simulink model "Final_big_controller"  (R2023b)
settings: Solver=VariableStepAuto  StartTime=0.0  StopTime=20  RelTol=1e-3
model workspace (MAT data in the model file):
  Kp_v = 1.5
  Kp_w = 6
settings Model: Creator=patel  LastModifiedBy=patel

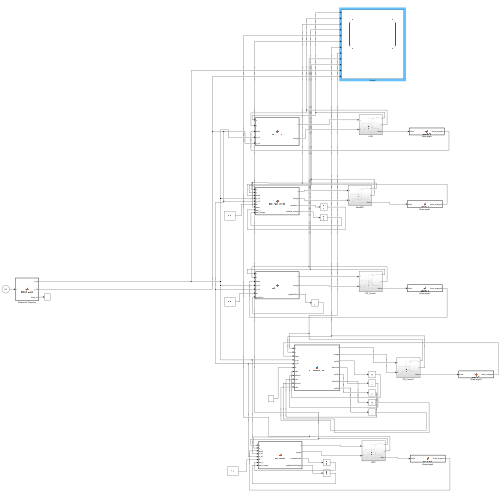
[thumbnail: Simulink's stored preview of the top-level diagram]
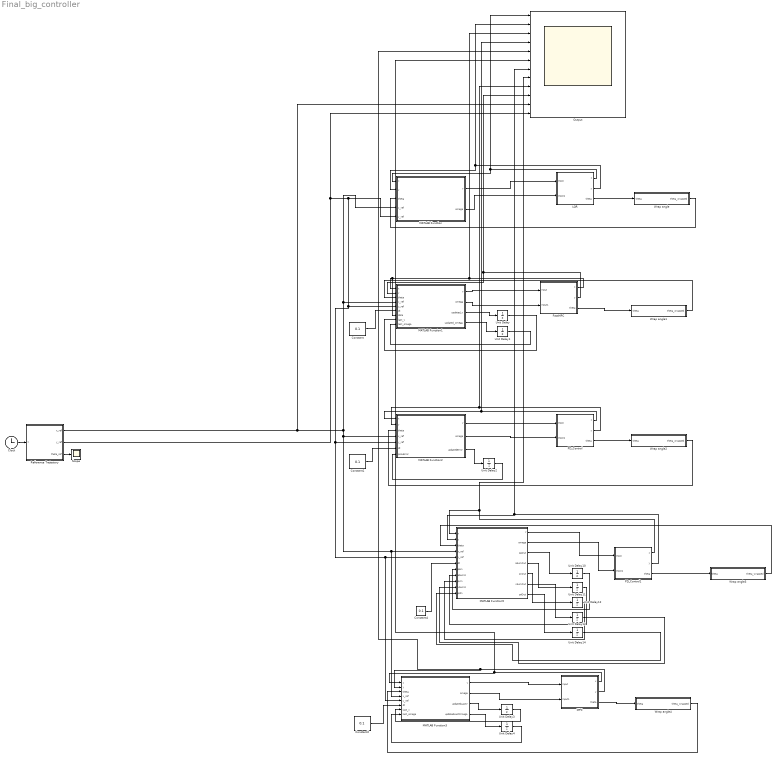
== system Final_big_controller ==
  Clock : Clock
      settings: Decimation=20
  Constant{,1..2,4} (4 alike) : Constant  Value=0.1
  FastMPC : Subsystem
  LQR : Subsystem
  MATLAB Function : MATLAB Function  TreatAsAtomicUnit=on
  MATLAB Function1 : MATLAB Function  TreatAsAtomicUnit=on
  MATLAB Function2 : MATLAB Function  TreatAsAtomicUnit=on
  MATLAB Function3 : MATLAB Function  TreatAsAtomicUnit=on
  MATLAB Function5 : MATLAB Function  TreatAsAtomicUnit=on
  MPC : Subsystem
  Output : Scope  NumInputPorts=12
  PD_Control : Subsystem
  PD_Control1 : Subsystem
  Reference Trajectory : MATLAB Function  TreatAsAtomicUnit=on
  Scope : Scope
  Unit Delay{,1..4,10..14} (10 alike) : UnitDelay  SampleTime=-1  HasFrameUpgradeWarning=on
  Wrap angle : MATLAB Function  TreatAsAtomicUnit=on
  Wrap angle1 : MATLAB Function  TreatAsAtomicUnit=on
  Wrap angle2 : MATLAB Function  TreatAsAtomicUnit=on
  Wrap angle3 : MATLAB Function  TreatAsAtomicUnit=on
  Wrap angle4 : MATLAB Function  TreatAsAtomicUnit=on
  wires:
  Reference Trajectory/3(theta_ref) -> Scope/1
  Clock/1 -> Reference Trajectory/1(t)
  MATLAB Function/2(omega) -> LQR/2(Input1)
  LQR/2(y) -> MATLAB Function/2(y), Output/2
  Wrap angle/1(theta_wrapped) -> MATLAB Function/3(theta)
  LQR/1(x) -> MATLAB Function/1(x), Output/1
  LQR/3(theta) -> Wrap angle/1(theta)
  MATLAB Function/1(v) -> LQR/1(Input)
  MATLAB Function1/4(updated_omega) -> Unit Delay1/1
  MATLAB Function1/3(updated_v) -> Unit Delay/1
  Constant/1 -> MATLAB Function1/6(dt)
  Unit Delay1/1 -> MATLAB Function1/9(last_omega)
  Unit Delay/1 -> MATLAB Function1/8(last_v)
  PD_Control/2(y) -> MATLAB Function2/2(y), Output/9
  MATLAB Function2/1(v) -> PD_Control/1(Input)
  Constant1/1 -> MATLAB Function2/6(dt)
  MATLAB Function2/2(omega) -> PD_Control/2(Input1)
  MATLAB Function2/3(updatedError) -> Unit Delay2/1
  PD_Control/1(x) -> Output/4, MATLAB Function2/1(x)
  Unit Delay2/1 -> MATLAB Function2/7(prevError)
  PD_Control1/1(x) -> MATLAB Function5/1(x), Output/8
  PD_Control1/2(y) -> Output/7, MATLAB Function5/2(y)
  Unit Delay4/1 -> MATLAB Function3/8(last_omega)
  Unit Delay3/1 -> MATLAB Function3/7(last_v)
  Reference Trajectory/2(y_ref) -> Output/12, MATLAB Function3/5(y_ref), MATLAB Function5/5(y_ref), MATLAB Function2/5(y_ref), MATLAB Function1/5(y_ref), MATLAB Function/5(y_ref)
  MPC/1(x) -> Output/6, MATLAB Function3/1(x)
  MPC/3(theta) -> Wrap angle4/1(theta)
  MATLAB Function3/3(updatedLastV) -> Unit Delay3/1
  Wrap angle4/1(theta_wrapped) -> MATLAB Function3/3(theta)
  MATLAB Function3/2(omega) -> MPC/2(Input1)
  Reference Trajectory/1(x_ref) -> Output/11, MATLAB Function/4(x_ref), MATLAB Function1/4(x_ref), MATLAB Function3/4(x_ref), MATLAB Function5/4(x_ref), MATLAB Function2/4(x_ref)
  MATLAB Function3/1(v) -> MPC/1(Input)
  MATLAB Function3/4(updatedLastOmega) -> Unit Delay4/1
  MPC/2(y) -> Output/5, MATLAB Function3/2(y)
  Constant2/1 -> MATLAB Function3/6(dt)
  MATLAB Function1/1(v) -> FastMPC/1(Input)
  MATLAB Function1/2(omega) -> FastMPC/2(Input1)
  FastMPC/3(theta) -> Wrap angle1/1(theta)
  Wrap angle1/1(theta_wrapped) -> MATLAB Function1/3(theta)
  FastMPC/1(x) -> Output/3, MATLAB Function1/7(data), MATLAB Function1/1(x)
  FastMPC/2(y) -> Output/10, MATLAB Function1/2(y)
  PD_Control/3(theta) -> Wrap angle2/1(theta)
  Wrap angle2/1(theta_wrapped) -> MATLAB Function2/3(theta)
  PD_Control1/3(theta) -> Wrap angle3/1(theta)
  MATLAB Function5/4(aSumOut) -> Unit Delay11/1
  Unit Delay14/1 -> MATLAB Function5/11(pdIn)
  MATLAB Function5/5(pvOut) -> Unit Delay12/1
  Constant4/1 -> MATLAB Function5/6(dt)
  Unit Delay12/1 -> MATLAB Function5/9(pvIn)
  Unit Delay13/1 -> MATLAB Function5/10(vSumIn)
  MATLAB Function5/6(vSumOut) -> Unit Delay13/1
  Unit Delay10/1 -> MATLAB Function5/7(paIn)
  Unit Delay11/1 -> MATLAB Function5/8(aSumIn)
  MATLAB Function5/3(paOut) -> Unit Delay10/1
  MATLAB Function5/7(pdOut) -> Unit Delay14/1
  MATLAB Function5/1(v) -> PD_Control1/1(Input)
  MATLAB Function5/2(omega) -> PD_Control1/2(Input1)
  Wrap angle3/1(theta_wrapped) -> MATLAB Function5/3(theta)

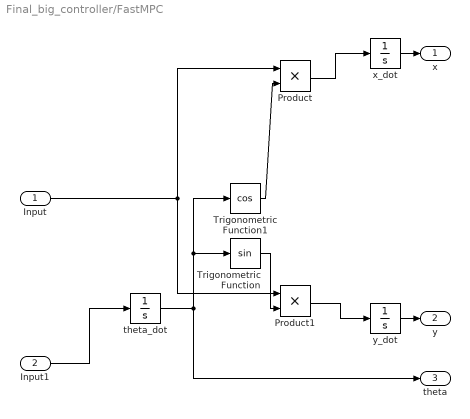
== system Final_big_controller/FastMPC ==
  Input : Inport
  Input1 : Inport  Port=2
  Product : Product
  Product1 : Product
  Trigonometric Function : Trigonometry
  Trigonometric Function1 : Trigonometry  Operator=cos
  theta_dot : Integrator
  x_dot : Integrator
  y_dot : Integrator
  x : Outport
  y : Outport  Port=2
  theta : Outport  Port=3
  wires:
  y_dot/1 -> y/1
  x_dot/1 -> x/1
  Product1/1 -> y_dot/1
  Trigonometric Function/1 -> Product1/2
  Input/1 -> Product/1, Product1/1
  Trigonometric Function1/1 -> Product/2
  Input1/1 -> theta_dot/1
  Product/1 -> x_dot/1
  theta_dot/1 -> Trigonometric Function/1, Trigonometric Function1/1, theta/1

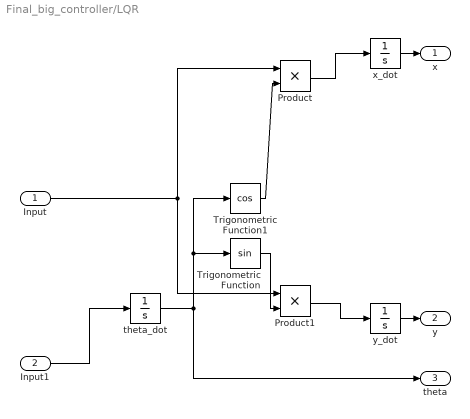
== system Final_big_controller/LQR ==
  Input : Inport
  Input1 : Inport  Port=2
  Product : Product
  Product1 : Product
  Trigonometric Function : Trigonometry
  Trigonometric Function1 : Trigonometry  Operator=cos
  theta_dot : Integrator
  x_dot : Integrator
  y_dot : Integrator
  x : Outport
  y : Outport  Port=2
  theta : Outport  Port=3
  wires:
  theta_dot/1 -> theta/1, Trigonometric Function1/1, Trigonometric Function/1
  Product/1 -> x_dot/1
  Input1/1 -> theta_dot/1
  Trigonometric Function1/1 -> Product/2
  Input/1 -> Product1/1, Product/1
  Trigonometric Function/1 -> Product1/2
  Product1/1 -> y_dot/1
  x_dot/1 -> x/1
  y_dot/1 -> y/1

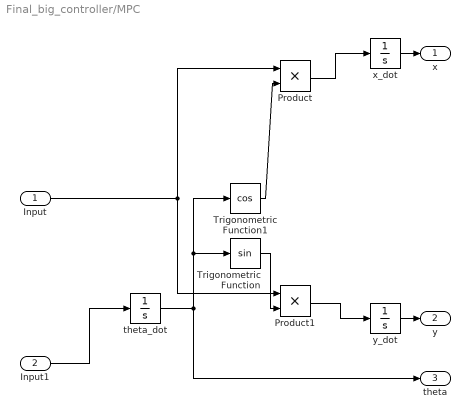
== system Final_big_controller/MPC ==
  Input : Inport
  Input1 : Inport  Port=2
  Product : Product
  Product1 : Product
  Trigonometric Function : Trigonometry
  Trigonometric Function1 : Trigonometry  Operator=cos
  theta_dot : Integrator
  x_dot : Integrator
  y_dot : Integrator
  x : Outport
  y : Outport  Port=2
  theta : Outport  Port=3
  wires:
  theta_dot/1 -> theta/1, Trigonometric Function1/1, Trigonometric Function/1
  Product/1 -> x_dot/1
  Input1/1 -> theta_dot/1
  Trigonometric Function1/1 -> Product/2
  Input/1 -> Product1/1, Product/1
  Trigonometric Function/1 -> Product1/2
  Product1/1 -> y_dot/1
  x_dot/1 -> x/1
  y_dot/1 -> y/1

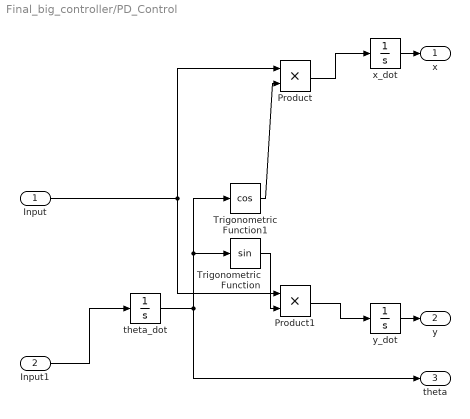
== system Final_big_controller/PD_Control ==
  Input : Inport
  Input1 : Inport  Port=2
  Product : Product
  Product1 : Product
  Trigonometric Function : Trigonometry
  Trigonometric Function1 : Trigonometry  Operator=cos
  theta_dot : Integrator
  x_dot : Integrator
  y_dot : Integrator
  x : Outport
  y : Outport  Port=2
  theta : Outport  Port=3
  wires:
  theta_dot/1 -> theta/1, Trigonometric Function1/1, Trigonometric Function/1
  Product/1 -> x_dot/1
  Input1/1 -> theta_dot/1
  Trigonometric Function1/1 -> Product/2
  Input/1 -> Product1/1, Product/1
  Trigonometric Function/1 -> Product1/2
  Product1/1 -> y_dot/1
  x_dot/1 -> x/1
  y_dot/1 -> y/1

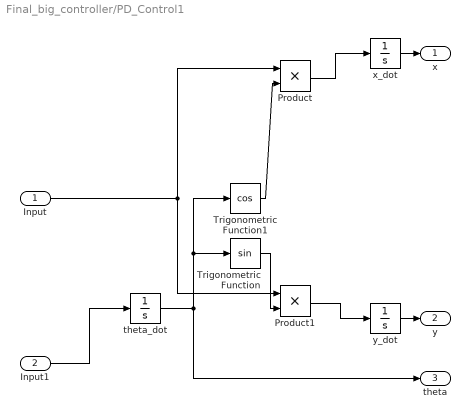
== system Final_big_controller/PD_Control1 ==
  Input : Inport
  Input1 : Inport  Port=2
  Product : Product
  Product1 : Product
  Trigonometric Function : Trigonometry
  Trigonometric Function1 : Trigonometry  Operator=cos
  theta_dot : Integrator
  x_dot : Integrator
  y_dot : Integrator
  x : Outport
  y : Outport  Port=2
  theta : Outport  Port=3
  wires:
  y_dot/1 -> y/1
  x_dot/1 -> x/1
  Product1/1 -> y_dot/1
  Trigonometric Function/1 -> Product1/2
  Input/1 -> Product/1, Product1/1
  Trigonometric Function1/1 -> Product/2
  Input1/1 -> theta_dot/1
  Product/1 -> x_dot/1
  theta_dot/1 -> Trigonometric Function/1, Trigonometric Function1/1, theta/1

== matlab function Final_big_controller/Wrap angle1 ==
  data: theta input; theta_wrapped output
function theta_wrapped = wrapToPi(theta)
    theta_wrapped = mod(theta + pi, 2*pi) - pi;
end

== matlab function Final_big_controller/Wrap angle2 ==
  data: theta input; theta_wrapped output
function theta_wrapped = wrapToPi(theta)
    theta_wrapped = mod(theta + pi, 2*pi) - pi;
end

== matlab function Final_big_controller/Wrap angle3 ==
  data: theta input; theta_wrapped output
function theta_wrapped = wrapToPi(theta)
    theta_wrapped = mod(theta + pi, 2*pi) - pi;
end

== matlab function Final_big_controller/Wrap angle4 ==
  data: theta input; theta_wrapped output
function theta_wrapped = wrapToPi(theta)
    theta_wrapped = mod(theta + pi, 2*pi) - pi;
end

== matlab function Final_big_controller/MATLAB Function5 ==
  data: x input; v output; y input; theta input; x_ref input; y_ref input; dt input; paIn input; aSumIn input; pvIn input; vSumIn input; pdIn input; omega output; paOut output; aSumOut output; pvOut output; vSumOut output; pdOut output
function [v, omega, paOut, aSumOut, pvOut, vSumOut, pdOut] = pid_controller_block(x, y, theta, x_ref, y_ref, dt, paIn, aSumIn, pvIn, vSumIn, pdIn)
%#codegen
robotState = [x; y; theta];
targetPoint = [x_ref; y_ref];
[v, omega, paOut, aSumOut, pvOut, vSumOut, pdOut] = PIDController(robotState, targetPoint, dt, paIn, aSumIn, pvIn, vSumIn, pdIn);

    function [v, omega, prevAngleError, angleErrorSum, prevVError, vErrorSum, prevDistance] = PIDController(robotState, targetPoint, dt, prevAngleError, angleErrorSum, prevVError, vErrorSum, prevDistance)
    % Unpack robot state
    x = robotState(1);
    y = robotState(2);
    theta = robotState(3);

    x_target = targetPoint(1);
    y_target = targetPoint(2);

    % Desired forward velocity
    v_desired = 5.0;

    %% --- Angular control (omega) ---
    angle_to_target = atan2(y_target - y, x_target - x);
    angle_error = atan2(sin(angle_to_target - theta), cos(angle_to_target - theta));
    angle_error_deriv = (angle_error - prevAngleError) / dt;
    angleErrorSum = angleErrorSum + angle_error * dt;
    angleErrorSum = min(max(angleErrorSum, -1.0), 1.0); % Anti-windup
    prevAngleError = angle_error;

    % PID gains for angular velocity
    kp_omega = 2.0;
    ki_omega = 1.0;
    kd_omega = 0.6;
    omega = kp_omega * angle_error + ki_omega * angleErrorSum + kd_omega * angle_error_deriv;
    omega = min(max(omega, -pi), pi);

    %% --- Linear velocity control ---
    dist_to_target = sqrt((x_target - x)^2 + (y_target - y)^2);
    v_current = (prevDistance - dist_to_target) / dt;
    prevDistance = dist_to_target;

    v_error = v_desired - v_current;
    v_error_deriv = (v_error - prevVError) / dt;
    vErrorSum = vErrorSum + v_error * dt;
    vErrorSum = min(max(vErrorSum, -2.0), 2.0); % Anti-windup
    prevVError = v_error;

    % PID gains for linear velocity
    kp_v = 1.0;
    ki_v = 0.5;
    kd_v = 0.2;
    v = kp_v * v_error + ki_v * vErrorSum + kd_v * v_error_deriv;

    % Reduce speed when not aligned with target
    v = v * cos(angle_error);

    % Clamp final velocity
    v = min(max(v, 0.2), 5.0);
end
    
end

== matlab function Final_big_controller/MATLAB Function1 ==
  data: x input; v output; y input; theta input; x_ref input; y_ref input; dt input; data input; last_v input; omega output; updated_v output; last_omega input; updated_omega output

function [v, omega, updated_v, updated_omega] = fast_mpc_control(x, y, theta, x_ref, y_ref, dt, data, last_v, last_omega)
%#codegen
robotState = [x; y; theta];
targetPoint = [x_ref; y_ref];
[v, omega, updated_v, updated_omega] = FastMPCController(robotState, targetPoint, dt, last_v, last_omega);

function [best_v, best_omega, last_v, last_omega] = FastMPCController(robotState, targetPoint, dt, last_v, last_omega)
    % Unpack current state
    x = robotState(1);
    y = robotState(2);
    theta = robotState(3);

    x_target = targetPoint(1);
    y_target = targetPoint(2);

    % MPC parameters
    N = 20;  % Prediction horizon

    % Cost weights (speed-prioritized)
    w_pos = 0.5;
    w_theta = 1.0;
    w_v = 0.05;
    w_omega = 0.1;
    velocity_bias = 0.3;  % Reward for high velocity

    % Control limits
    v_min = 0.0;
    v_max = 5.0;
    omega_min = -pi;
    omega_max = pi;

    % Control search ranges (favoring acceleration)
    v_range_min = max(v_min, last_v - 0.3);
    v_range_max = min(v_max, last_v + 0.7);
    v_options = linspace(v_range_min, v_range_max, 5);
    omega_options = linspace(max(omega_min, last_omega - 0.5), min(omega_max, last_omega + 0.5), 7);

    % Initialize best control
    best_cost = inf;
    best_v = last_v;
    best_omega = last_omega;

    for vi = 1:length(v_options)
        for wi = 1:length(omega_options)
            v = v_options(vi);
            omega = omega_options(wi);

            pred_x = x;
            pred_y = y;
            pred_theta = theta;
            total_cost = 0;

            for i = 0:N-1
                % Predict next state
                pred_x = pred_x + v * cos(pred_theta) * dt;
                pred_y = pred_y + v * sin(pred_theta) * dt;
                pred_theta = pred_theta + omega * dt;

                % Errors
                pos_error = sqrt((x_target - pred_x)^2 + (y_target - pred_y)^2);
                desired_theta = atan2(y_target - pred_y, x_target - pred_x);
                theta_error = atan2(sin(desired_theta - pred_theta), cos(desired_theta - pred_theta));

                % Smoothness
                v_change = abs(v - last_v);
                omega_change = abs(omega - last_omega);

                % Reward for speed
                velocity_reward = -velocity_bias * v / v_max;

                % Step cost
                step_cost = w_pos * pos_error + w_theta * abs(theta_error) + w_v * v_change + w_omega * omega_change + velocity_reward;
                discount = 0.9 ^ i;
                total_cost = total_cost + discount * step_cost;
            end

            % Update best control
            if total_cost < best_cost
                best_cost = total_cost;
                best_v = v;
                best_omega = omega;
            end
        end
    end

    % Update memory for next call
    last_v = best_v;
    last_omega = best_omega;
end
end

== matlab function Final_big_controller/Reference Trajectory ==
  data: t input; x_ref output; y_ref output; theta_ref output
function [x_ref, y_ref, theta_ref] = trajectoryGen(t)
    radius = 5;
    omega_ref = 0.2;
    x_ref = radius * cos(omega_ref * t);
    y_ref = radius * sin(omega_ref * t);
    theta_ref = omega_ref * t + pi/2;
end

== matlab function Final_big_controller/Wrap angle ==
  data: theta input; theta_wrapped output
function theta_wrapped = wrapToPi(theta)
    theta_wrapped = mod(theta + pi, 2*pi) - pi;
end

== matlab function Final_big_controller/MATLAB Function ==
  data: x input; v output; y input; theta input; x_ref input; y_ref input; omega output
function [v, omega] = lqr_control(x, y, theta, x_ref, y_ref)
%#codegen
robotState = [x; y; theta];
targetPoint = [x_ref; y_ref];
[v, omega] = LQRController(robotState, targetPoint);

function [v, omega] = LQRController(robotState, targetPoint)
    % Inputs:
    %   robotState = [x; y; theta]
    %   targetPoint = [x_target; y_target]

    x = robotState(1);
    y = robotState(2);
    theta = robotState(3);

    x_target = targetPoint(1);
    y_target = targetPoint(2);

    % LQR Gain matrix (2x3)
    K = [1.5, 0.0, 0.0;
         0.0, 1.5, 2.0];

    % Global error
    dx = x_target - x;
    dy = y_target - y;
    error_global = [dx; dy];

    % Rotation matrix to robot frame
    c = cos(theta);
    s = sin(theta);
    R = [c, s; -s, c];
    error_robot = R * error_global;

    % Theta error
    angle_to_target = atan2(dy, dx);
    theta_error = atan2(sin(angle_to_target - theta), cos(angle_to_target - theta));

    % Form error state
    error_state = [error_robot; theta_error];

    % Control input via LQR gains
    v_r = K(1, :) * error_state;
    v_l = K(2, :) * error_state;

    % Convert to unicycle model control inputs
    v = (v_r + v_l) / 2;
    omega = (v_r - v_l) / 0.2;  % 0.2m wheel base

    % Saturation
    v = max(0.2, min(v, 5.0));
    omega = min(max(omega, -pi), pi);
end
end

== matlab function Final_big_controller/MATLAB Function2 ==
  data: x input; v output; y input; theta input; x_ref input; y_ref input; dt input; prevError input; omega output; updatedError output

function [v, omega, updatedError] = pd_control(x, y, theta, x_ref, y_ref, dt, prevError)
%#codegen
robotState = [x; y; theta];
targetPoint = [x_ref; y_ref];
[v, omega, updatedError] = PD_Controller(robotState, targetPoint, dt, prevError);

    function [v, omega, updatedPrevAngleError] = PD_Controller(robotState, targetPoint, dt, prevAngleError)
    x = robotState(1); y = robotState(2); theta = robotState(3);
    x_target = targetPoint(1); y_target = targetPoint(2);

    dx = x_target - x;
    dy = y_target - y;
    dist_to_target = sqrt(dx^2 + dy^2);

    angle_to_target = atan2(dy, dx);
    angle_error = atan2(sin(angle_to_target - theta), cos(angle_to_target - theta));
    angle_error_deriv = (angle_error - prevAngleError) / dt;
    updatedPrevAngleError = angle_error;

    % PD Gains
    kp_v = 1.5;
    kp_omega = 2.0;
    kd_omega = 1.0;

    v = min(max(kp_v * dist_to_target, 0.2), 5.0);
    omega = min(max(kp_omega * angle_error + kd_omega * angle_error_deriv, -pi), pi);
end

end

== matlab function Final_big_controller/MATLAB Function3 ==
  data: x input; v output; y input; theta input; x_ref input; y_ref input; dt input; last_v input; omega output; updatedLastV output; last_omega input; updatedLastOmega output

function [v, omega, updatedLastV, updatedLastOmega] = mpc_control(x, y, theta, x_ref, y_ref, dt, last_v, last_omega)
%#codegen
robotState = [x; y; theta];
targetPoint = [x_ref; y_ref];
[v, omega, updatedLastV, updatedLastOmega] = MPCController(robotState, targetPoint, dt, last_v, last_omega);

function [best_v, best_omega, last_v, last_omega] = MPCController(robotState, targetPoint, dt, last_v, last_omega)
    % Unpack state
    x = robotState(1);
    y = robotState(2);
    theta = robotState(3);
    
    x_target = targetPoint(1);
    y_target = targetPoint(2);

    % MPC Parameters
    N = 10;  % Prediction horizon

    % Weights
    w_pos = 1.0;
    w_theta = 1.5;
    w_v = 0.1;
    w_omega = 0.2;

    % Control limits
    v_min = 0.2; v_max = 5.0;
    omega_min = -pi; omega_max = pi;

    % Discretized control space
    v_options = linspace(max(v_min, last_v - 0.5), min(v_max, last_v + 0.5), 5);
    omega_options = linspace(max(omega_min, last_omega - 0.5), min(omega_max, last_omega + 0.5), 7);

    % Initialize best control
    best_cost = inf;
    best_v = last_v;
    best_omega = last_omega;

    % Evaluate control sequences
    for vi = 1:length(v_options)
        for wi = 1:length(omega_options)
            v = v_options(vi);
            omega = omega_options(wi);

            pred_x = x;
            pred_y = y;
            pred_theta = theta;
            total_cost = 0;

            for i = 0:N-1
                % Predict next state
                pred_x = pred_x + v * cos(pred_theta) * dt;
                pred_y = pred_y + v * sin(pred_theta) * dt;
                pred_theta = pred_theta + omega * dt;

                % Compute errors
                pos_error = sqrt((x_target - pred_x)^2 + (y_target - pred_y)^2);
                desired_theta = atan2(y_target - pred_y, x_target - pred_x);
                theta_error = atan2(sin(desired_theta - pred_theta), cos(desired_theta - pred_theta));

                % Control smoothness
                v_change = abs(v - last_v);
                omega_change = abs(omega - last_omega);

                % Cost with discount
                step_cost = w_pos * pos_error + w_theta * abs(theta_error) + w_v * v_change + w_omega * omega_change;
                discount = 0.9 ^ i;
                total_cost = total_cost + discount * step_cost;
            end

            % Update best control
            if total_cost < best_cost
                best_cost = total_cost;
                best_v = v;
                best_omega = omega;
            end
        end
    end

    % Update memory for next step
    last_v = best_v;
    last_omega = best_omega;
end

end
